simulink model "New_specific_volume"  (R2013b)
settings: Solver=FixedStepDiscrete  StartTime=0.0  StopTime=0  FixedStep=1  RelTol=1e-3
libraries: carnot x1
settings Model: DEBUGGLOBALLEVEL=1  DEBUGWRITETOFILE=0  DEBUGFILENAME=bla.txt  DEBUGMAXCONSECUTIVEWARNINGS=inf  DEBUGMAXTOTALWARNINGS=inf  Creator=awohlfei  LastModifiedBy=awohlfei
settings OptimizationCC: ExpressionDepthLimit=2147483647
settings DebuggingCC: UnderspecifiedInitializationDetection=Simplified  MergeDetectMultiDrivingBlocksExec=error  StateNameClashWarn=warning

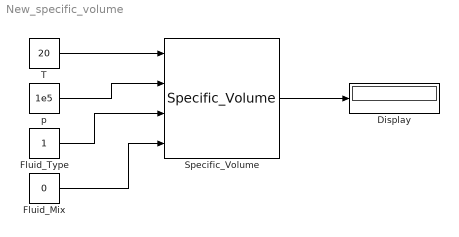
== system New_specific_volume ==
  Display : Display
  Fluid_Mix : Constant  Value=0
  Fluid_Type : Constant
  Specific_Volume : carnot/Basic/Material_Properties/Specific_Volume  VariantControl=CarlibClassic  INPUTARGUMENTS=state variables (classic)  DEBUGLEVEL=DEBUGLEVEL  MAXTOTALWARNINGS=inf  MAXCONSECUTIVEWARNINGS=inf  WRITETOFILE=0  FILENAME='errors.txt'
  T : Constant  Value=20
  p : Constant  Value=1e5
  wires:
  T/1 -> Specific_Volume/1
  p/1 -> Specific_Volume/2
  Fluid_Mix/1 -> Specific_Volume/4
  Specific_Volume/1 -> Display/1
  Fluid_Type/1 -> Specific_Volume/3
